simulink model "s_track_model"  (R2023b)
settings: Solver=ode4  StartTime=0.0  StopTime=t_end_sim  FixedStep=dt_sim  RelTol=1e-3  EnableMultiTasking=on
undefined symbols (not defined in the file): A_sim, B_sim, C_sim, D_sim, delta_vol_max_ramp, dvol_drift1, dvol_drift2, dvol_drift3, dvol_max, sel_man, t_drift_cs_1, t_drift_cs_2, t_end_sim, tau_s, V
libraries: simulink_extras x6, simulink x4
settings Model: Creator=gianl  LastModifiedBy=dadog
settings SolverCC: AlgebraicLoopSolver=TrustRegion
settings DataIOCC: ReturnWorkspaceOutputs=off
settings OptimizationCC: LifeSpan=1
settings DebuggingCC: UnconnectedInputMsg=warning  UnconnectedOutputMsg=warning  UnconnectedLineMsg=warning  SFExecutionAtInitializationDiag=none  ArithmeticOperatorsInVariantConditions=warning
settings ModelReferenceCC: EnableRefExpFcnMdlSchedulingChecks=on
settings SFSimCC: SimUseLocalCustomCode=off  CustomCodeUndefinedFunction=UseInterfaceOnly
settings RTWCC: RTWUseLocalCustomCode=off  DLArmComputeVersion=19.05
settings CodeAppCC: StateflowObjectComments=on

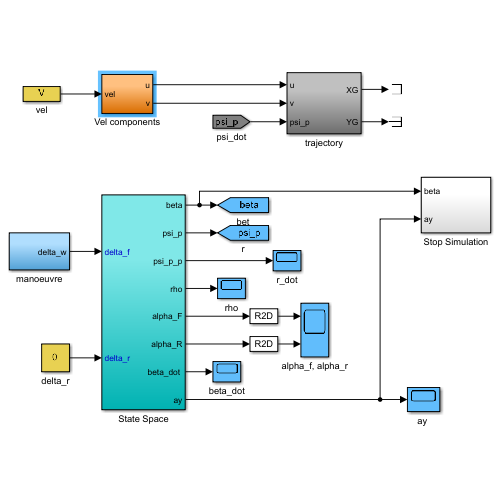
[thumbnail: Simulink's stored preview of the top-level diagram]
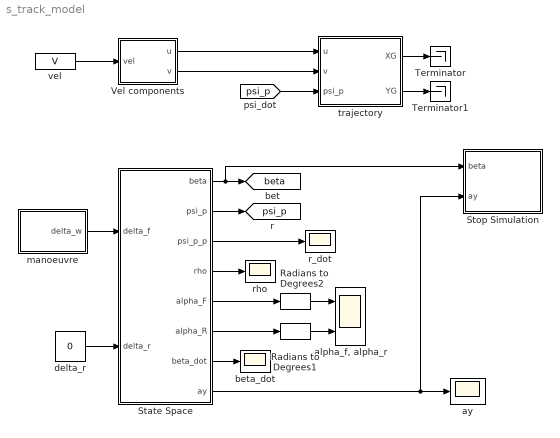
== system s_track_model ==
  Radians to Degrees1 : simulink_extras/Transformations/Radians to Degrees
  Radians to Degrees2 : simulink_extras/Transformations/Radians to Degrees
  State Space : Subsystem
  Stop Simulation : Subsystem
  Terminator : Terminator
  Terminator1 : Terminator
  Vel components : Subsystem
  "alpha_f, alpha_r" : Scope  NumInputPorts=2
  "ay " : Scope
  beta_dot : Scope
  delta_r : Constant  Value=0
  manoeuvre : Subsystem
  r_dot : Scope
  rho : Scope
  trajectory : Subsystem
  vel : Constant  Value=V
  tag scope: beta=global, psi_p=global
  wires:
  manoeuvre/1(delta_w) -> State Space/1(delta_f)
  State Space/1(beta) -> [beta], Stop Simulation/1(beta)
  State Space/2(psi_p) -> [psi_p]
  State Space/3(psi_p_p) -> r_dot/1
  vel/1 -> Vel components/1(vel)
  Vel components/1(u) -> trajectory/1(u)
  Vel components/2(v) -> trajectory/2(v)
  [psi_p] -> trajectory/3(psi_p)
  State Space/4(rho) -> rho/1
  State Space/5(alpha_F) -> Radians to Degrees2/1
  State Space/6(alpha_R) -> Radians to Degrees1/1
  trajectory/1(XG) -> Terminator/1
  trajectory/2(YG) -> Terminator1/1
  delta_r/1 -> State Space/2(delta_r)
  State Space/7("beta_dot ") -> beta_dot/1
  State Space/8(ay) -> Stop Simulation/2(ay), "ay "/1
  Radians to Degrees2/1 -> "alpha_f, alpha_r"/1
  Radians to Degrees1/1 -> "alpha_f, alpha_r"/2

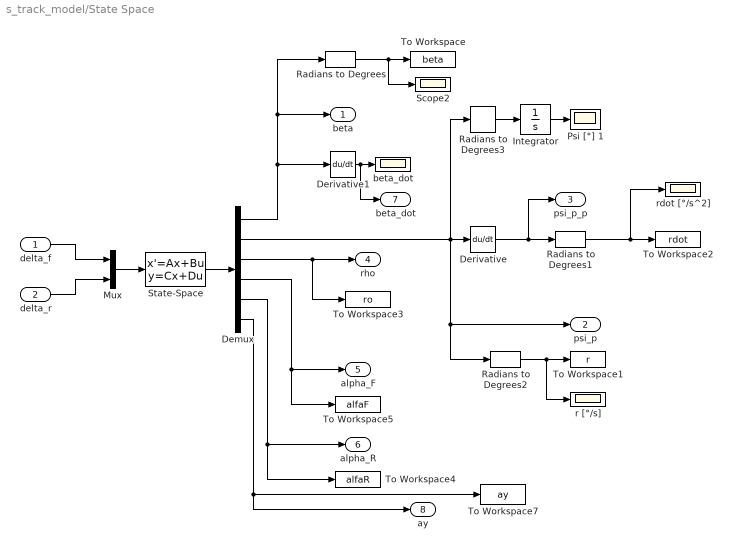
== system s_track_model/State Space ==
  delta_f : Inport
  delta_r : Inport  Port=2
  Demux : Demux  Outputs=6
  Derivative : Derivative
  Derivative1 : Derivative
  Integrator : Integrator
  Mux : Mux  Inputs=2
  Psi [°] 1 : Scope
  Radians to Degrees{,1..3} (4 alike) : simulink_extras/Transformations/Radians to Degrees
  Scope2 : Scope
  State-Space : StateSpace  A=A_sim  B=B_sim  C=C_sim  D=D_sim  InitialCondition=0
  To Workspace : ToWorkspace  VariableName=beta  SaveFormat=Timeseries  SampleTime=-1
  To Workspace1 : ToWorkspace  VariableName=r  SaveFormat=Timeseries  SampleTime=-1
  To Workspace2 : ToWorkspace  VariableName=rdot  SaveFormat=Timeseries  SampleTime=-1
  To Workspace3 : ToWorkspace  VariableName=ro  SaveFormat=Timeseries  SampleTime=-1
  To Workspace4 : ToWorkspace  VariableName=alfaR  SaveFormat=Timeseries  SampleTime=-1
  To Workspace5 : ToWorkspace  VariableName=alfaF  SaveFormat=Timeseries  SampleTime=-1
  To Workspace7 : ToWorkspace  VariableName=ay  SaveFormat=Timeseries  SampleTime=-1
      settings: Save2DSignal=2-D array (concatenate along first dimension)
  beta_dot : Scope
  r [°/s] : Scope
  rdot [°/s^2] : Scope
  beta : Outport  VectorParamsAs1DForOutWhenUnconnected=off
  psi_p : Outport  Port=2  VectorParamsAs1DForOutWhenUnconnected=off
  psi_p_p : Outport  Port=3  VectorParamsAs1DForOutWhenUnconnected=off
  rho : Outport  Port=4  VectorParamsAs1DForOutWhenUnconnected=off
  alpha_F : Outport  Port=5  VectorParamsAs1DForOutWhenUnconnected=off
  alpha_R : Outport  Port=6  VectorParamsAs1DForOutWhenUnconnected=off
  "beta_dot " : Outport  Port=7  VectorParamsAs1DForOutWhenUnconnected=off
  ay : Outport  Port=8  VectorParamsAs1DForOutWhenUnconnected=off
  wires:
  Demux/2 -> psi_p/1, Radians to Degrees2/1, Radians to Degrees3/1, Derivative/1
  Demux/1 -> Derivative1/1, beta/1, Radians to Degrees/1
  Derivative/1 -> Radians to Degrees1/1, psi_p_p/1
  Radians to Degrees/1 -> Scope2/1, To Workspace/1
  Radians to Degrees1/1 -> rdot [°/s^2]/1, To Workspace2/1
  Radians to Degrees2/1 -> r [°/s]/1, To Workspace1/1
  Demux/3 -> To Workspace3/1, rho/1
  Demux/4 -> alpha_F/1, To Workspace5/1
  Demux/5 -> To Workspace4/1, alpha_R/1
  Radians to Degrees3/1 -> Integrator/1
  Integrator/1 -> Psi [°] 1/1
  Derivative1/1 -> "beta_dot "/1, beta_dot/1
  delta_f/1 -> Mux/1
  delta_r/1 -> Mux/2
  Demux/6 -> ay/1, To Workspace7/1
  Mux/1 -> State-Space/1
  State-Space/1 -> Demux/1

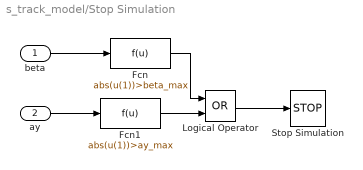
== system s_track_model/Stop Simulation ==
  beta : Inport
  ay : Inport  Port=2
  Fcn : Fcn  Expr=abs(u(1))>beta_max
  Fcn1 : Fcn  Expr=abs(u(1))>ay_max
  Logical Operator : Logic  Operator=OR  AllPortsSameDT=off  OutDataTypeStr=boolean
  Stop Simulation : Stop
  wires:
  Logical Operator/1 -> Stop Simulation/1
  ay/1 -> Fcn1/1
  beta/1 -> Fcn/1
  Fcn1/1 -> Logical Operator/2
  Fcn/1 -> Logical Operator/1

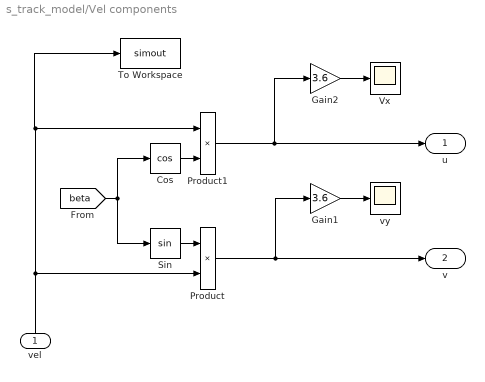
== system s_track_model/Vel components ==
  vel : Inport
  Cos : Trigonometry  Operator=cos
  Gain1 : Gain  Gain=3.6
  Gain2 : Gain  Gain=3.6
  Product : Product
  Product1 : Product
  Sin : Trigonometry
  To Workspace : ToWorkspace  VariableName=simout  SaveFormat=Timeseries  SampleTime=-1
  Vx : Scope
  vy : Scope
  u : Outport  VectorParamsAs1DForOutWhenUnconnected=off
  v : Outport  Port=2  VectorParamsAs1DForOutWhenUnconnected=off
  wires:
  Product/1 -> Gain1/1, v/1
  vel/1 -> Product/2, Product1/1, To Workspace/1
  Gain1/1 -> vy/1
  Gain2/1 -> Vx/1
  Cos/1 -> Product1/2
  Product1/1 -> Gain2/1, u/1
  [beta] -> Sin/1, Cos/1
  Sin/1 -> Product/1

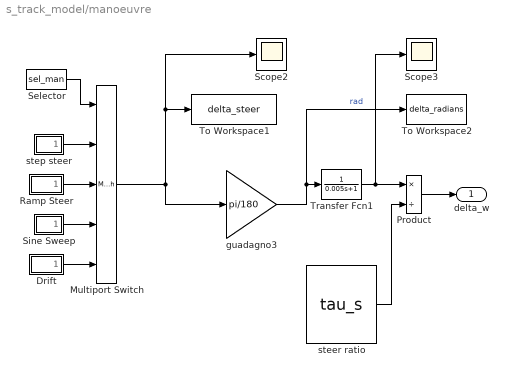
== system s_track_model/manoeuvre ==
  Drift : Subsystem
  Multiport Switch : MultiPortSwitch  Inputs=4  SaturateOnIntegerOverflow=off  InputSameDT=off
  Product : Product  Inputs=*/  RndMeth=Zero
  Ramp Steer : Subsystem
  Scope2 : Scope
  Scope3 : Scope
  Selector : Constant  Value=sel_man
  Sine Sweep : Subsystem
  To Workspace1 : ToWorkspace  VariableName=delta_steer  SaveFormat=Timeseries  SampleTime=-1
  To Workspace2 : ToWorkspace  VariableName=delta_radians  SaveFormat=Timeseries  SampleTime=-1
  Transfer Fcn1 : TransferFcn  Denominator=[0.005 1]
  guadagno3 : Gain  Gain=pi/180  SaturateOnIntegerOverflow=on  OutDataTypeStr=Inherit: Same as input  ParamDataTypeStr=Inherit: Same as input
  "steer ratio " : Constant  Value=tau_s
  step steer : Subsystem
  delta_w : Outport  VectorParamsAs1DForOutWhenUnconnected=off
  wires:
  Selector/1 -> Multiport Switch/1
  Ramp Steer/1(delta) -> Multiport Switch/3
  step steer/1(delta) -> Multiport Switch/2
  Multiport Switch/1 -> guadagno3/1, To Workspace1/1, Scope2/1
  guadagno3/1 -> To Workspace2/1, Transfer Fcn1/1  "rad"
  "steer ratio "/1 -> Product/2
  Product/1 -> delta_w/1
  Transfer Fcn1/1 -> Scope3/1, Product/1
  Sine Sweep/1(delta) -> Multiport Switch/4
  Drift/1(delta) -> Multiport Switch/5

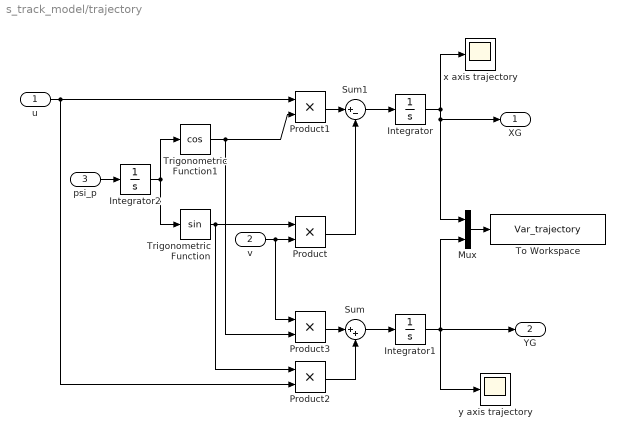
== system s_track_model/trajectory ==
  u : Inport
  v : Inport  Port=2
  psi_p : Inport  Port=3
  Integrator : Integrator
  Integrator1 : Integrator
  Integrator2 : Integrator
  Mux : Mux  Inputs=2
  Product{,1..3} (4 alike) : Product  InputSameDT=on  SaturateOnIntegerOverflow=on  OutDataTypeStr=Inherit: Same as first input
  Sum : Sum  Inputs=|++  InputSameDT=on  SaturateOnIntegerOverflow=on  OutDataTypeStr=Inherit: Same as first input
  Sum1 : Sum  Inputs=|+-  InputSameDT=on  SaturateOnIntegerOverflow=on  OutDataTypeStr=Inherit: Same as first input
  To Workspace : ToWorkspace  VariableName=Var_trajectory  SampleTime=-1
      settings: Save2DSignal=2-D array (concatenate along first dimension)
      settings: InitFcn=|
      | ParentName = get_param(gcb,'Parent');
      | cont = max(find(ParentName=='/'));
      | set_param(gcb,'VariableName',strcat('Var_',ParentName(cont+1:length(ParentName))));
      | clear ParentName cont
  Trigonometric Function : Trigonometry
  Trigonometric Function1 : Trigonometry  Operator=cos
  x axis trajectory : Scope
  y axis trajectory : Scope
  XG : Outport  VectorParamsAs1DForOutWhenUnconnected=off
  YG : Outport  Port=2  VectorParamsAs1DForOutWhenUnconnected=off
  wires:
  psi_p/1 -> Integrator2/1
  Product1/1 -> Sum1/1
  Product/1 -> Sum1/2
  Sum1/1 -> Integrator/1
  Trigonometric Function/1 -> Product/1, Product2/1
  u/1 -> Product2/2, Product1/1
  v/1 -> Product/2, Product3/1
  Trigonometric Function1/1 -> Product1/2, Product3/2
  Product3/1 -> Sum/1
  Product2/1 -> Sum/2
  Sum/1 -> Integrator1/1
  Integrator/1 -> XG/1, Mux/1, x axis trajectory/1
  Integrator1/1 -> YG/1, y axis trajectory/1, Mux/2
  Mux/1 -> To Workspace/1
  Integrator2/1 -> Trigonometric Function/1, Trigonometric Function1/1

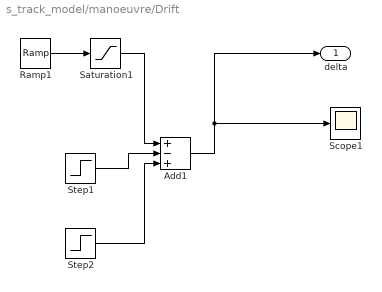
== system s_track_model/manoeuvre/Drift ==
  Add1 : Sum  Inputs=+-+
  Ramp1 : simulink/Sources/Ramp  slope=400  start=1  InitialOutput=0
  Saturation1 : Saturate  UpperLimit=dvol_drift1  LowerLimit=0
  Scope1 : Scope
  Step1 : Step  Time=t_drift_cs_1  After=dvol_drift2  SampleTime=0
  Step2 : Step  Time=t_drift_cs_2  After=dvol_drift3  SampleTime=0
  delta : Outport  VectorParamsAs1DForOutWhenUnconnected=off
  wires:
  Step2/1 -> Add1/3
  Saturation1/1 -> Add1/1
  Add1/1 -> delta/1, Scope1/1
  Step1/1 -> Add1/2
  Ramp1/1 -> Saturation1/1

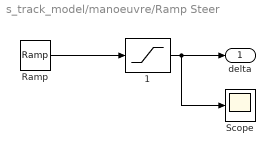
== system s_track_model/manoeuvre/Ramp Steer ==
  "  1" : Saturate  UpperLimit=delta_vol_max_ramp  LowerLimit=-delta_vol_max_ramp
  Ramp : simulink/Sources/Ramp  slope=15  start=1  InitialOutput=0
  Scope : Scope
  delta : Outport  VectorParamsAs1DForOutWhenUnconnected=off
  wires:
  "  1"/1 -> Scope/1, delta/1
  Ramp/1 -> "  1"/1

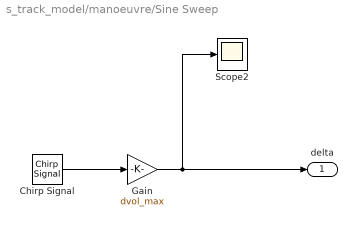
== system s_track_model/manoeuvre/Sine Sweep ==
  Chirp Signal : simulink/Sources/Chirp Signal  f1=0.01  T=t_end_sim  f2=5
  Gain : Gain  Gain=dvol_max
  Scope2 : Scope
  delta : Outport  InitialOutput=0  VectorParamsAs1DForOutWhenUnconnected=off
  wires:
  Chirp Signal/1 -> Gain/1
  Gain/1 -> delta/1, Scope2/1

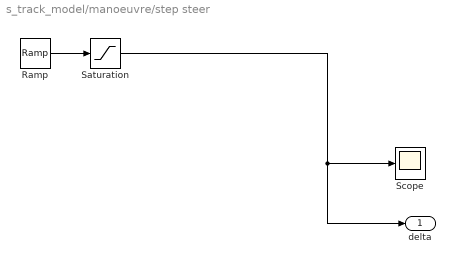
== system s_track_model/manoeuvre/step steer ==
  Ramp : simulink/Sources/Ramp  slope=400  start=1  InitialOutput=0
  Saturation : Saturate  UpperLimit=dvol_max  LowerLimit=0
  Scope : Scope
  delta : Outport  VectorParamsAs1DForOutWhenUnconnected=off
  wires:
  Ramp/1 -> Saturation/1
  Saturation/1 -> delta/1, Scope/1
